simulink model "exercise12b"  (R2018b)
settings: Solver=VariableStepAuto  StartTime=0.0  StopTime=10.0  RelTol=1e-3
settings Model: Creator=Alireza  LastModifiedBy=Alireza

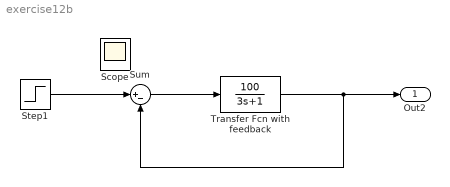
== system exercise12b ==
  Step1 : Step  SampleTime=0
  Sum : Sum  Inputs=|+-
  Transfer Fcn with feedback : TransferFcn  Numerator=[100]  Denominator=[3 1]
  Out2 : Outport
  Scope : Scope
  wires:
  Transfer Fcn with feedback/1 -> Sum/2, Out2/1
  Step1/1 -> Sum/1
  Sum/1 -> Transfer Fcn with feedback/1
